simulink model "figura_1"  (R2021b)
settings: Solver=ode23t  StartTime=0.0  StopTime=0.1  RelTol=1e-5
libraries: spsCurrentMeasurementLib x2, spsGroundLib x2, spsThreePhaseSourceLib x1, spsFourierLib x1, spsThreePhaseSeriesRLCBranchLib x1, spsPowerLib x1, spsVoltageMeasurementLib x1, spspowerguiLib x1
settings Model: Creator=alanp  LastModifiedBy=luang
settings SolverCC: AlgebraicLoopSolver=TrustRegion
settings DebuggingCC: SFMachineParentedDataDiag=warning

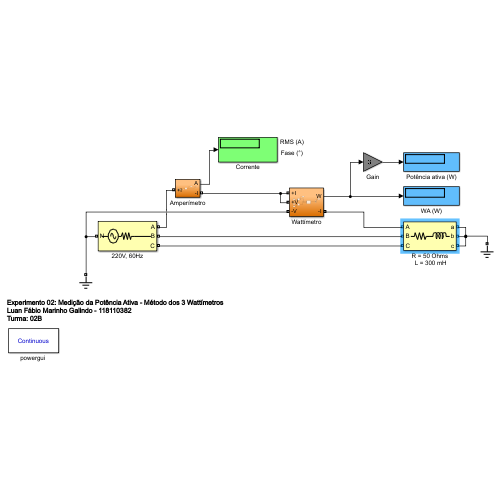
[thumbnail: Simulink's stored preview of the top-level diagram]
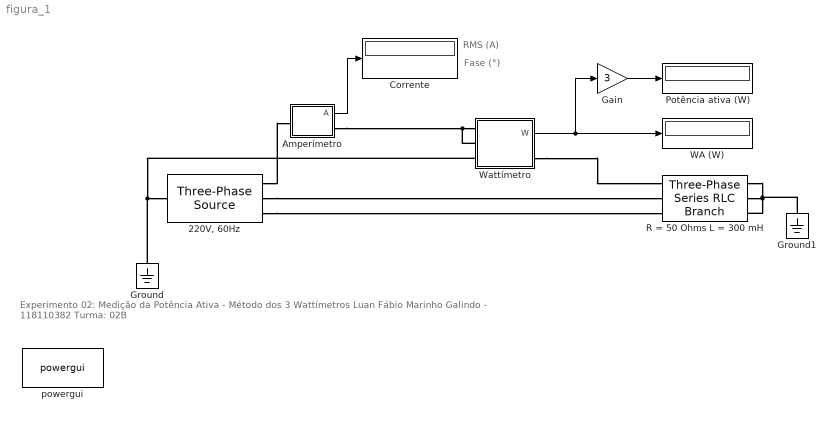
== system figura_1 ==
  note: Fase (°)
  note: RMS (A)
  note: Experimento 02: Medição da Potência Ativa - Método dos 3 Wattímetros
      | Luan Fábio Marinho Galindo - 118110382
      | Turma: 02B
  "220V, 60Hz" : spsThreePhaseSourceLib/Three-Phase Source  InternalConnection=Yn  VoltagePhases=off  Voltage=220  PhaseAngle=90  Voltage_phases=[25e3 25e3 25e3]/sqrt(3)  PhaseAngles_phases=[0 -120 +120]  Frequency=60  NonIdealSource=on  SpecifyImpedance=off  Resistance=0.001  Inductance=0  ShortCircuitLevel=100e6  BaseVoltage=25e3  XRratio=7  BusType=swing  Pref=10e3  Qref=0  Prefabc=[10e3, 10e3, 10e3]  Qrefabc=[0, 0, 0]  Qmin=-inf  Qmax=inf
  Amperímetro : Subsystem
  Corrente : Display
      settings: Format=bank
  Gain : Gain  Gain=3
  Ground : spsGroundLib/Ground  LConnTagsString=a
  Ground1 : spsGroundLib/Ground  LConnTagsString=a
  Potência ativa (W) : Display
      settings: Format=bank
  R = 50 Ohms L = 300 mH : spsThreePhaseSeriesRLCBranchLib/Three-Phase Series RLC Branch  LConnTagsString=A|B|C  RConnTagsString=A|B|C  BranchType=RL  Resistance=50  Inductance=300e-3  Capacitance=0  Measurements=None
  WA (W) : Display
      settings: Format=bank
  Wattímetro : Subsystem
  "powergui " : spspowerguiLib/powergui  Priority=1  SimulationMode=Continuous  SampleTime=50e-6  frequency=60  Iterations=50  frequencyindice=60  Pbase=100e6  ErrMax=1e-4  UnitsV=kV  UnitsW=MW  buscounter=0  FunctionMessages=off  echomessages=off  EnableUseOfTLC=off  CurrentSourceSwitches=off  DisableSnubberDevices=off  DisableRonSwitches=off  DisableVfSwitches=off  DisplayEquations=off  AutomaticDiscreteSolvers=off  SolverType=Tustin/Backward Euler (TBE)  Interpol=off  ExternalGateDelay=off  methode=off  Ts=100  x0status=blocks  SPID=on  SwTol=0  HookPort=off  NonlinearTolerance=1e-4  nMaxIteration=100  ContinueOnMaxIteration=off  RestoreLinks=warning  ResistiveCurrentMeasurement=off  Frange=[0:2:500]  Ylog=off  Xlog=on  ShowGrid=off  save=off  variable=ZData  structure=0  ZoomFFT=off  StartTime=0.0  cycles=1  DisplayStyle=1  fundamental=60  FreqAxis=off  MaxFrequency=1000  frequencyindicesteady=1  RmsSteady=1  display=off
  wires:
  Wattímetro/1(W) -> Gain/1, WA (W)/1
  Gain/1 -> Potência ativa (W)/1
  Amperímetro/1(A) -> Corrente/1
  connections:
  Ground/LConn1 -- Wattímetro/LConn3 -- "220V, 60Hz"/LConn1
  "220V, 60Hz"/RConn2 -- R = 50 Ohms L = 300 mH/LConn2
  "220V, 60Hz"/RConn3 -- R = 50 Ohms L = 300 mH/LConn3
  R = 50 Ohms L = 300 mH/RConn1 -- Ground1/LConn1 -- R = 50 Ohms L = 300 mH/RConn2 -- R = 50 Ohms L = 300 mH/RConn3
  Wattímetro/RConn1 -- R = 50 Ohms L = 300 mH/LConn1
  "220V, 60Hz"/RConn1 -- Amperímetro/LConn1
  Amperímetro/RConn1 -- Wattímetro/LConn2 -- Wattímetro/LConn1

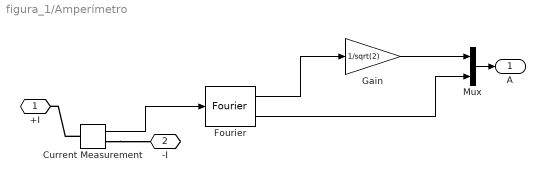
== system figura_1/Amperímetro ==
  Current Measurement : spsCurrentMeasurementLib/Current Measurement  PhasorSimulation=off  OutputType=Complex  PSBequivalent=0
  Fourier : spsFourierLib/Fourier  Freq=60  n=1  InInit=[0, 0]  Ts=0
      settings: SourceProductBaseCode=PS
  Gain : Gain  Gain=1/sqrt(2)
  Mux : Mux  Inputs=2
  +I : PMIOPort  Side=Left
  -I : PMIOPort  Port=2  Side=Right
  A : Outport
  wires:
  Gain/1 -> Mux/1
  Fourier/1 -> Gain/1
  Mux/1 -> A/1
  Fourier/2 -> Mux/2
  Current Measurement/1 -> Fourier/1
  connections:
  Current Measurement/RConn1 -- -I/RConn1
  Current Measurement/LConn1 -- +I/RConn1

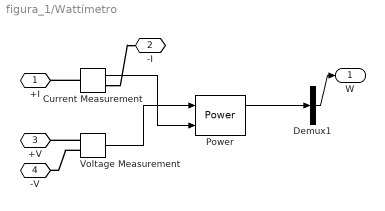
== system figura_1/Wattímetro ==
  Current Measurement : spsCurrentMeasurementLib/Current Measurement  PhasorSimulation=off  OutputType=Complex  PSBequivalent=0
  Demux1 : Demux  Outputs=1
  Power : spsPowerLib/Power  Freq=60  Vinit=[1, 0]  Iinit=[1, 0]  Ts=0
      settings: SourceProductBaseCode=PS
  Voltage Measurement : spsVoltageMeasurementLib/Voltage Measurement  PhasorSimulation=off  OutputType=Complex  PSBequivalent=0
  +I : PMIOPort  Side=Left
  -I : PMIOPort  Port=2  Side=Right
  +V : PMIOPort  Port=3  Side=Left
  -V : PMIOPort  Port=4  Side=Left
  W : Outport
  wires:
  Current Measurement/1 -> Power/2
  Power/1 -> Demux1/1
  Demux1/1 -> W/1
  Voltage Measurement/1 -> Power/1
  connections:
  Voltage Measurement/LConn1 -- +V/RConn1
  Voltage Measurement/LConn2 -- -V/RConn1
  Current Measurement/LConn1 -- +I/RConn1
  Current Measurement/RConn1 -- -I/RConn1
